simulink model "pd_nf_pi"  (R2023a)
settings: Solver=VariableStepAuto  StartTime=0.0  StopTime=10.0  RelTol=1e-3
values from neighbouring files (symbols this model uses):
  h_g_z : value not decoded    [dictionary_srf_pll.sldd]
  NF_z2 : value not decoded    [dictionary_srf_pll.sldd]
  tsample = 0.0002    [dictionary_srf_pll.sldd]
settings Model: DataDictionary=dictionary.sldd  Creator=ASUSTUF  LastModifiedBy=ASUSTUF

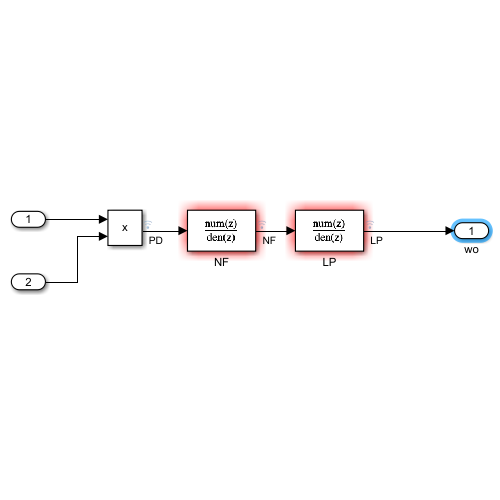
[thumbnail: Simulink's stored preview of the top-level diagram]
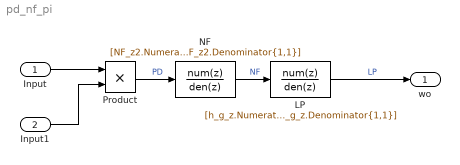
== system pd_nf_pi ==
  Input : Inport
  Input1 : Inport  Port=2
  LP : DiscreteTransferFcn  Numerator=[h_g_z.Numerator{1,1}]  Denominator=[h_g_z.Denominator{1,1}]  SampleTime=tsample  OutDataTypeStr=fixdt(1,32,24)
  NF : DiscreteTransferFcn  Numerator=[NF_z2.Numerator{1,1}]  Denominator=[NF_z2.Denominator{1,1}]  SampleTime=tsample  OutDataTypeStr=fixdt(1,32,31)
  Product : Product
  wo : Outport
  wires:
  Input1/1 -> Product/2
  Input/1 -> Product/1
  LP/1 -> wo/1  "LP"
  NF/1 -> LP/1  "NF"
  Product/1 -> NF/1  "PD"
